simulink model "Modele_detaille_2019a"  (R2023a)
settings: Solver=VariableStepAuto  StartTime=0.0  StopTime=10.0  RelTol=1e-3
undefined symbols (not defined in the file): i0, k1, k2, Ki, Kz, Te, z0
libraries: dspsrcs4 x1
settings Model: Creator=xshi  LastModifiedBy=leolebuhotel
settings SolverCC: AlgebraicLoopSolver=TrustRegion
settings OptimizationCC: ReuseModelBlockBuffer=off
settings DebuggingCC: UnconnectedInputMsg=warning  UnconnectedOutputMsg=warning  UnconnectedLineMsg=warning
settings ModelReferenceCC: EnableRefExpFcnMdlSchedulingChecks=on
settings SFSimCC: CustomCodeUndefinedFunction=UseInterfaceOnly

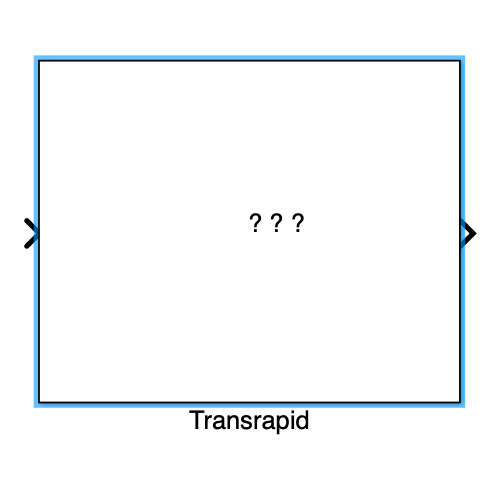
[thumbnail: Simulink's stored preview of the top-level diagram]
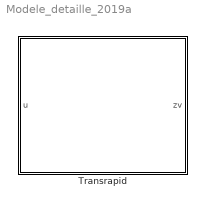
== system Modele_detaille_2019a ==
  Transrapid : Subsystem
      mask Display:
      | image('Transrapid.jpg');
      | color('yellow')
      | port_label('output', 1, 'z');
      | port_label('input', 1, 'commande u');

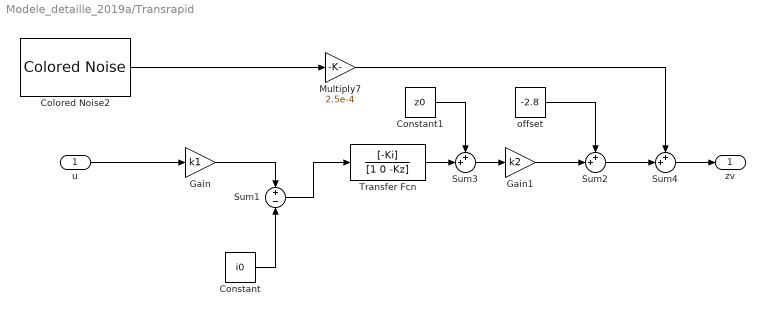
== system Modele_detaille_2019a/Transrapid ==
  u : Inport
  Colored Noise2 : dspsrcs4/Colored Noise  Color=white  InverseFrequencyPower=1  NumChannels=1  OutputDataType=double  SamplesPerFrame=1  SampleTime=Te  RandomStream=mt19937ar with seed  Seed=67  SimulateUsing=Interpreted execution
  Constant : Constant  Value=i0
  Constant1 : Constant  Value=z0
  Gain : Gain  Gain=k1
  Gain1 : Gain  Gain=k2
  Multiply7 : Gain  Gain=2.5e-4
  Sum1 : Sum  Inputs=+-
  Sum2 : Sum  Inputs=++|
  Sum3 : Sum  Inputs=++|
  Sum4 : Sum  Inputs=++|
  Transfer Fcn : TransferFcn  Numerator=[-Ki]  Denominator=[1 0 -Kz]
  offset : Constant  Value=-2.8
  zv : Outport
  wires:
  Sum3/1 -> Gain1/1
  Transfer Fcn/1 -> Sum3/2
  Gain/1 -> Sum1/1
  Constant/1 -> Sum1/2
  Sum1/1 -> Transfer Fcn/1
  Constant1/1 -> Sum3/1
  Gain1/1 -> Sum2/2
  offset/1 -> Sum2/1
  Sum2/1 -> Sum4/2
  Sum4/1 -> zv/1
  Multiply7/1 -> Sum4/1
  Colored Noise2/1 -> Multiply7/1
  u/1 -> Gain/1
